simulink library "xps_library"  (R2021a)
settings: Solver=VariableStepAuto  StartTime=0.0  StopTime=10.0  RelTol=1e-3
undefined symbols (not defined in the file): ip_name, lib_path
libraries: xbsIndex_r4 x2612, casper_library_flow_control x68, simulink x52, $bdroot x9, casper_library_misc x9
(part 1 of 35)
settings Model: Creator=jkocz  LastModifiedBy=casperlwa

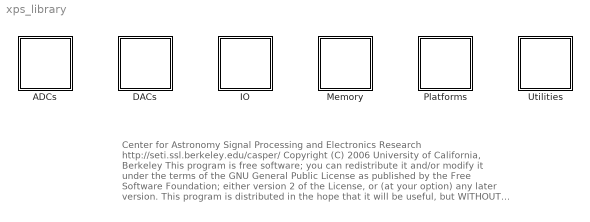
== system xps_library ==
  note: Center for Astronomy Signal Processing and Electronics Research
      | http://seti.ssl.berkeley.edu/casper/
      | Copyright (C) 2006 University of California, Berkeley
      |
      | This program is free software; you can redistribute it and/or modify
      | it under the terms of the GNU General Public License as published by
      | the Free Software Foundation; either version 2 of the License, or
      | (at your option) any later version.
      |
      | This program is distributed in the hope that it will be useful,
      | but WITHOUT ANY WARRANTY; without even the implied warranty of
      | MERCHANTABILITY or FITNESS FOR A PARTICULAR PURPOSE.  See the
      | GNU General Public License for more details.
      |
      | You should have received a copy of the GNU General Public License along
      | with this program; if not, write to the Free Software Foundation, Inc.,
      | 51 Franklin Street, Fifth Floor, Boston, MA 02110-1301 USA.
  ADCs : Subsystem  Tag=group
  DACs : Subsystem  Tag=group
  IO : Subsystem  Tag=group
  Memory : Subsystem  Tag=group
  Platforms : Subsystem  Tag=group
  Utilities : Subsystem  Tag=group
